simulink library "SimscapeCustomComponents_lib"  (R2025b)
settings: Solver=VariableStepAuto  StartTime=0.0  StopTime=10.0  RelTol=1e-3
undefined symbols (not defined in the file or in its folder): base, baseVdc, capacity, DiscIntNeverNeededParam, ee_sli_rtmsupport, filterInductance, freqeuncy, frequency, gcbh, gflInverter, gfmInverter, iMaxPU, Inertia, initialSOC, plantRating, solar, Ts, ups, Vac, windSystem, windTurbine
libraries: fl_lib x397, nesl_utility x171, eeGeneralControl x85, ee_lib x82, simulink x72, datacenter_lib x68, eeTransforms x38, slpidlib x24, buildingEnergy_lib x20, SimscapeFluids_lib x17, eeSinusoidalMeasurementV2 x8, eePwmGenerator x8
(part 10 of 24)

== system SimscapeCustomComponents_lib/Microgrid and Renewables/Control/Microgrid/Black Start ==
  Enable : Inport  OutDataTypeStr=boolean
  Voltage : Inport  Port=2  OutDataTypeStr=boolean
  Abs : Abs  SaturateOnIntegerOverflow=off
  Constant : Constant  Value=0.05
  Constant1 : Constant  Value=voltageLevel1+voltageLevel2+voltageLevel3
  Data Type Conversion : DataTypeConversion  OutDataTypeStr=double  SaturateOnIntegerOverflow=off  RndMeth=Floor
  Data Type Conversion1 : DataTypeConversion  OutDataTypeStr=boolean  SaturateOnIntegerOverflow=off  RndMeth=Floor
  Delay : Delay  DelayLength=10
  Frequency Reference : Subsystem
  Gain : Gain
  LessThanOrEqual : RelationalOperator  Operator=<=  OutDataTypeStr=boolean  RndMeth=Simplest  InputSameDT=off
  Product : Product
  Subtract : Sum  Inputs=+-
  Voltage Reference : Subsystem
  Status : Outport
  Bus Element Out2 : Outport  Port=2  PortName=BlackStart  Element=Vref
  Bus Element Out3 : Outport  Port=2  PortName=BlackStart  Element=Fref
  Bus Element Out1 : Outport  Port=2  PortName=BlackStart  Element=enableCommand
  wires:
  Voltage Reference/1(VRef) -> Bus Element Out2/1
  Data Type Conversion/1 -> Gain/1
  Data Type Conversion1/1 -> Status/1
  Enable/1 -> Voltage Reference/1(Enable), Data Type Conversion/1
  Delay/1 -> Product/1
  Abs/1 -> LessThanOrEqual/1
  Constant1/1 -> Subtract/2
  Product/1 -> Data Type Conversion1/1
  Voltage/1 -> Subtract/1
  Constant/1 -> LessThanOrEqual/2
  LessThanOrEqual/1 -> Product/2
  Frequency Reference/1(FRef) -> Bus Element Out3/1
  Subtract/1 -> Abs/1
  Gain/1 -> Bus Element Out1/1, Delay/1

== system SimscapeCustomComponents_lib/Microgrid and Renewables/Control/Microgrid/PlannedIslanding ==
  Enable : Inport
  P : Inport  Port=2
  Q : Inport  Port=3
  Data Type Conversion : DataTypeConversion  OutDataTypeStr=double  SaturateOnIntegerOverflow=off  RndMeth=Floor
  Logical Operator : Logic  AllPortsSameDT=off  OutDataTypeStr=boolean
  PID Frequency : slpidlib/PID Controller  Controller=PI  Form=Parallel  TimeDomain=Discrete-time  UseExternalTs=off  SampleTime=Ts  IntegratorMethod=Forward Euler  FilterMethod=Forward Euler  ControllerParametersSource=internal  P=KpPPlannedIsland  I=KiPPlannedIsland  UseKiTs=off  D=0  UseExternalDerivativeSource=off  N=100  UseFilter=on  TunerSelectOption=Frequency Response Based  InitialConditionSource=internal  InitialConditionForIntegrator=0  InitialConditionForFilter=0  DifferentiatorICPrevScaledInput=0  ExternalReset=none  TrackingMode=off  Kt=1  LimitOutput=off  SatLimitsSource=internal  UpperSaturationLimit=0.05  LowerSaturationLimit=-0.05  LinearizeAsGain=on  AntiWindupMode=clamping  Kb=1  LimitIntegrator=off  UpperIntegratorSaturationLimit=inf  LowerIntegratorSaturationLimit=-inf  POutMin=[]  POutMax=[]  IOutMin=[]  IOutMax=[]  DOutMin=[]  DOutMax=[]  NOutMin=[]  NOutMax=[]  SumOutMin=[]  SumOutMax=[]  SaturationOutMin=[]  SaturationOutMax=[]  PParamMin=[]  PParamMax=[]  IParamMin=[]  IParamMax=[]  DParamMin=[]  DParamMax=[]  NParamMin=[]  NParamMax=[]  KbParamMin=[]  KbParamMax=[]  KtParamMin=[]  KtParamMax=[]  KbOutMin=[]  KbOutMax=[]  KtOutMin=[]  KtOutMax=[]  IntegratorOutMin=[]  IntegratorOutMax=[]  FilterOutMin=[]  FilterOutMax=[]  SumI1OutMin=[]  SumI1OutMax=[]  SumI2OutMin=[]  SumI2OutMax=[]  SumI3OutMin=[]  SumI3OutMax=[]  SumI4OutMin=[]  SumI4OutMax=[]  SumDOutMin=[]  SumDOutMax=[]  DifferentiatorOutMin=[]  DifferentiatorOutMax=[]  FilterDiffOutCoefMin=[]  FilterDiffOutCoefMax=[]  ReciprocalOutMin=[]  ReciprocalOutMax=[]  SumDenOutMin=[]  SumDenOutMax=[]  SumNumOutMin=[]  SumNumOutMax=[]  DivideOutMin=[]  DivideOutMax=[]  UdiffTsProdOutMin=[]  UdiffTsProdOutMax=[]  NTsProdOutMin=[]  NTsProdOutMax=[]  UintegralTsProdOutMin=[]  UintegralTsProdOutMax=[]  UngainTsProdOutMin=[]  UngainTsProdOutMax=[]  ClampingZeroOutDataTypeStr=Inherit: Inherit via back propagation  ClampingZeroOutMin=[]  ClampingZeroOutMax=[]  FilterDenConstantOutDataTypeStr=Inherit: Inherit via back propagation  FilterDenConstantOutMin=[]  FilterDenConstantOutMax=[]  PCopyOutDataTypeStr=Inherit: Inherit via back propagation  PCopyOutMin=[]  PCopyOutMax=[]  NCopyOutDataTypeStr=Inherit: Inherit via back propagation  NCopyOutMin=[]  NCopyOutMax=[]  IntegratorContinuousStateAttributes=''  IntegratorStateMustResolveToSignalObject=off  IntegratorRTWStateStorageClass=Auto  FilterContinuousStateAttributes=''  FilterStateMustResolveToSignalObject=off  FilterRTWStateStorageClass=Auto  ParallelPVariant=InternalParameters  IdealPVariant=Disabled  IVariant=InternalParameters  DVariant=Disabled  IntegratorVariant=Discrete  SatVariant=Disabled  AWVariant=Passthrough  PCopyVariant=Disabled  TRVariant=Disabled  FdbkBlocksVariant=Forward  IdealPFdbkVariant=Disabled  SatFdbkVariant=Disabled  DerivativeFilterVariant=Disabled  NVariant=Disabled  NCopyVariant=Disabled_SignalSpec  FilterICVariant=Disabled  IntegratorICVariant=InternalICs  ExternalResetVariant=Disabled  TRSumVariant=Passthrough  SumFdbkVariant=Disabled  SumVariant=Sum_PI  TsampFilterVariant=InternalTs  TsampNgainVariant=Passthrough  TsampIntegralVariant=Disabled_SignalSpec  ExternalSaturationOutDataTypeStr=Inherit: Same as second input  DerivativeSourceVariant=Disabled  PreIntVariant=InternalPreInt
  PID voltage : slpidlib/PID Controller  Controller=PI  Form=Parallel  TimeDomain=Discrete-time  UseExternalTs=off  SampleTime=Ts  IntegratorMethod=Forward Euler  FilterMethod=Forward Euler  ControllerParametersSource=internal  P=KpQPlannedIsland  I=KiQPlannedIsland  UseKiTs=off  D=0  UseExternalDerivativeSource=off  N=100  UseFilter=on  TunerSelectOption=Frequency Response Based  InitialConditionSource=internal  InitialConditionForIntegrator=0  InitialConditionForFilter=0  DifferentiatorICPrevScaledInput=0  ExternalReset=none  TrackingMode=off  Kt=1  LimitOutput=off  SatLimitsSource=internal  UpperSaturationLimit=0.05  LowerSaturationLimit=-0.05  LinearizeAsGain=on  AntiWindupMode=clamping  Kb=1  LimitIntegrator=off  UpperIntegratorSaturationLimit=inf  LowerIntegratorSaturationLimit=-inf  POutMin=[]  POutMax=[]  IOutMin=[]  IOutMax=[]  DOutMin=[]  DOutMax=[]  NOutMin=[]  NOutMax=[]  SumOutMin=[]  SumOutMax=[]  SaturationOutMin=[]  SaturationOutMax=[]  PParamMin=[]  PParamMax=[]  IParamMin=[]  IParamMax=[]  DParamMin=[]  DParamMax=[]  NParamMin=[]  NParamMax=[]  KbParamMin=[]  KbParamMax=[]  KtParamMin=[]  KtParamMax=[]  KbOutMin=[]  KbOutMax=[]  KtOutMin=[]  KtOutMax=[]  IntegratorOutMin=[]  IntegratorOutMax=[]  FilterOutMin=[]  FilterOutMax=[]  SumI1OutMin=[]  SumI1OutMax=[]  SumI2OutMin=[]  SumI2OutMax=[]  SumI3OutMin=[]  SumI3OutMax=[]  SumI4OutMin=[]  SumI4OutMax=[]  SumDOutMin=[]  SumDOutMax=[]  DifferentiatorOutMin=[]  DifferentiatorOutMax=[]  FilterDiffOutCoefMin=[]  FilterDiffOutCoefMax=[]  ReciprocalOutMin=[]  ReciprocalOutMax=[]  SumDenOutMin=[]  SumDenOutMax=[]  SumNumOutMin=[]  SumNumOutMax=[]  DivideOutMin=[]  DivideOutMax=[]  UdiffTsProdOutMin=[]  UdiffTsProdOutMax=[]  NTsProdOutMin=[]  NTsProdOutMax=[]  UintegralTsProdOutMin=[]  UintegralTsProdOutMax=[]  UngainTsProdOutMin=[]  UngainTsProdOutMax=[]  ClampingZeroOutDataTypeStr=Inherit: Inherit via back propagation  ClampingZeroOutMin=[]  ClampingZeroOutMax=[]  FilterDenConstantOutDataTypeStr=Inherit: Inherit via back propagation  FilterDenConstantOutMin=[]  FilterDenConstantOutMax=[]  PCopyOutDataTypeStr=Inherit: Inherit via back propagation  PCopyOutMin=[]  PCopyOutMax=[]  NCopyOutDataTypeStr=Inherit: Inherit via back propagation  NCopyOutMin=[]  NCopyOutMax=[]  IntegratorContinuousStateAttributes=''  IntegratorStateMustResolveToSignalObject=off  IntegratorRTWStateStorageClass=Auto  FilterContinuousStateAttributes=''  FilterStateMustResolveToSignalObject=off  FilterRTWStateStorageClass=Auto  ParallelPVariant=InternalParameters  IdealPVariant=Disabled  IVariant=InternalParameters  DVariant=Disabled  IntegratorVariant=Discrete  SatVariant=Disabled  AWVariant=Passthrough  PCopyVariant=Disabled  TRVariant=Disabled  FdbkBlocksVariant=Forward  IdealPFdbkVariant=Disabled  SatFdbkVariant=Disabled  DerivativeFilterVariant=Disabled  NVariant=Disabled  NCopyVariant=Disabled_SignalSpec  FilterICVariant=Disabled  IntegratorICVariant=InternalICs  ExternalResetVariant=Disabled  TRSumVariant=Passthrough  SumFdbkVariant=Disabled  SumVariant=Sum_PI  TsampFilterVariant=InternalTs  TsampNgainVariant=Passthrough  TsampIntegralVariant=Disabled_SignalSpec  ExternalSaturationOutDataTypeStr=Inherit: Same as second input  DerivativeSourceVariant=Disabled  PreIntVariant=InternalPreInt
  Planned Island Time Delay : Subsystem
  Product{,1..3} (4 alike) : Product
  Scope : Scope  NumInputPorts=2
      settings: ActiveDisplayYMinimum=-1  ActiveDisplayYMaximum=1  DataLoggingVariableName=ScopeData35
  Scope1 : Scope  NumInputPorts=2
      settings: ActiveDisplayYMinimum=-1.6827967094302978  ActiveDisplayYMaximum=1.1685546180291482  DataLoggingVariableName=ScopeData36
  Subsystem : Subsystem
  Subsystem1 : Subsystem
  Status : Outport
  Bus Element Out : Outport  Port=2  PortName=PlannedIslanding  Element=enableCommand
  BusElementOut : Outport  Port=2  PortName=PlannedIslanding  Element=activePower
  BusElementOut1 : Outport  Port=2  PortName=PlannedIslanding  Element=reactivePower
  BusElementOut2 : Outport  Port=2  PortName=PlannedIslanding  Element=status
  wires:
  Product1/1 -> Subsystem/1(AVTIVE POWER ERROR), PID Frequency/1
  Product3/1 -> Logical Operator/2
  PID voltage/1 -> Scope/2, BusElementOut1/1
  [plannedIslanding] -> Product3/1
  [plannedIslanding] -> Planned Island Time Delay/2(In2)
  [plannedIslanding] -> Product/1
  PID Frequency/1 -> BusElementOut/1, Scope/1
  Planned Island Time Delay/1(Status) -> BusElementOut2/1, Status/1
  Product/1 -> Logical Operator/1
  Q/1 -> Scope1/2, Product2/2
  Subsystem1/1(Out1) -> Product3/2
  [plannedIslanding] -> Product1/2, Product2/1
  Subsystem/1(Out1) -> Product/2
  P/1 -> Scope1/1, Product1/1
  Logical Operator/1 -> Planned Island Time Delay/1(In1)
  Enable/1 -> Data Type Conversion/1
  Product2/1 -> PID voltage/1, Subsystem1/1(REACTIVEPOWER ERROR)
  Data Type Conversion/1 -> Bus Element Out/1, [plannedIslanding]
  ? -> ?

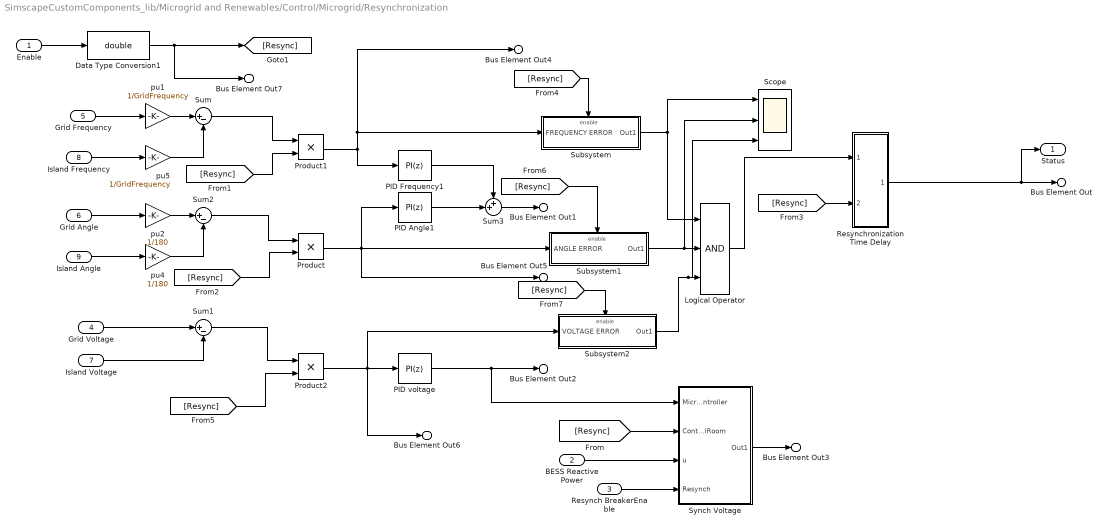
== system SimscapeCustomComponents_lib/Microgrid and Renewables/Control/Microgrid/Resynchronization ==
  Enable : Inport  OutDataTypeStr=double
  BESS Reactive Power : Inport  Port=2
  Resynch BreakerEnable : Inport  Port=3
  Grid Voltage : Inport  Port=4
  Grid Frequency : Inport  Port=5
  Grid Angle : Inport  Port=6
  Island Voltage : Inport  Port=7
  Island Frequency : Inport  Port=8
  Island Angle : Inport  Port=9
  Data Type Conversion1 : DataTypeConversion  OutDataTypeStr=double  SaturateOnIntegerOverflow=off  RndMeth=Floor
  Logical Operator : Logic  Inputs=3  AllPortsSameDT=off  OutDataTypeStr=boolean
  PID Angle1 : slpidlib/PID Controller  Controller=PI  Form=Parallel  TimeDomain=Discrete-time  UseExternalTs=off  SampleTime=Ts  IntegratorMethod=Forward Euler  FilterMethod=Forward Euler  ControllerParametersSource=internal  P=KpAngResynch  I=KiAngResynch  UseKiTs=off  D=0  UseExternalDerivativeSource=off  N=100  UseFilter=on  TunerSelectOption=Frequency Response Based  InitialConditionSource=internal  InitialConditionForIntegrator=0  InitialConditionForFilter=0  DifferentiatorICPrevScaledInput=0  ExternalReset=none  TrackingMode=off  Kt=1  LimitOutput=off  SatLimitsSource=internal  UpperSaturationLimit=0.5  LowerSaturationLimit=-0.5  LinearizeAsGain=on  AntiWindupMode=clamping  Kb=1  LimitIntegrator=off  UpperIntegratorSaturationLimit=inf  LowerIntegratorSaturationLimit=-inf  POutMin=[]  POutMax=[]  IOutMin=[]  IOutMax=[]  DOutMin=[]  DOutMax=[]  NOutMin=[]  NOutMax=[]  SumOutMin=[]  SumOutMax=[]  SaturationOutMin=[]  SaturationOutMax=[]  PParamMin=[]  PParamMax=[]  IParamMin=[]  IParamMax=[]  DParamMin=[]  DParamMax=[]  NParamMin=[]  NParamMax=[]  KbParamMin=[]  KbParamMax=[]  KtParamMin=[]  KtParamMax=[]  KbOutMin=[]  KbOutMax=[]  KtOutMin=[]  KtOutMax=[]  IntegratorOutMin=[]  IntegratorOutMax=[]  FilterOutMin=[]  FilterOutMax=[]  SumI1OutMin=[]  SumI1OutMax=[]  SumI2OutMin=[]  SumI2OutMax=[]  SumI3OutMin=[]  SumI3OutMax=[]  SumI4OutMin=[]  SumI4OutMax=[]  SumDOutMin=[]  SumDOutMax=[]  DifferentiatorOutMin=[]  DifferentiatorOutMax=[]  FilterDiffOutCoefMin=[]  FilterDiffOutCoefMax=[]  ReciprocalOutMin=[]  ReciprocalOutMax=[]  SumDenOutMin=[]  SumDenOutMax=[]  SumNumOutMin=[]  SumNumOutMax=[]  DivideOutMin=[]  DivideOutMax=[]  UdiffTsProdOutMin=[]  UdiffTsProdOutMax=[]  NTsProdOutMin=[]  NTsProdOutMax=[]  UintegralTsProdOutMin=[]  UintegralTsProdOutMax=[]  UngainTsProdOutMin=[]  UngainTsProdOutMax=[]  ClampingZeroOutDataTypeStr=Inherit: Inherit via back propagation  ClampingZeroOutMin=[]  ClampingZeroOutMax=[]  FilterDenConstantOutDataTypeStr=Inherit: Inherit via back propagation  FilterDenConstantOutMin=[]  FilterDenConstantOutMax=[]  PCopyOutDataTypeStr=Inherit: Inherit via back propagation  PCopyOutMin=[]  PCopyOutMax=[]  NCopyOutDataTypeStr=Inherit: Inherit via back propagation  NCopyOutMin=[]  NCopyOutMax=[]  IntegratorContinuousStateAttributes=''  IntegratorStateMustResolveToSignalObject=off  IntegratorRTWStateStorageClass=Auto  FilterContinuousStateAttributes=''  FilterStateMustResolveToSignalObject=off  FilterRTWStateStorageClass=Auto  ParallelPVariant=InternalParameters  IdealPVariant=Disabled  IVariant=InternalParameters  DVariant=Disabled  IntegratorVariant=Discrete  SatVariant=Disabled  AWVariant=Passthrough  PCopyVariant=Disabled  TRVariant=Disabled  FdbkBlocksVariant=Forward  IdealPFdbkVariant=Disabled  SatFdbkVariant=Disabled  DerivativeFilterVariant=Disabled  NVariant=Disabled  NCopyVariant=Disabled_SignalSpec  FilterICVariant=Disabled  IntegratorICVariant=InternalICs  ExternalResetVariant=Disabled  TRSumVariant=Passthrough  SumFdbkVariant=Disabled  SumVariant=Sum_PI  TsampFilterVariant=InternalTs  TsampNgainVariant=Passthrough  TsampIntegralVariant=Disabled_SignalSpec  ExternalSaturationOutDataTypeStr=Inherit: Same as second input  DerivativeSourceVariant=Disabled  PreIntVariant=InternalPreInt
  PID Frequency1 : slpidlib/PID Controller  Controller=PI  Form=Parallel  TimeDomain=Discrete-time  UseExternalTs=off  SampleTime=Ts  IntegratorMethod=Forward Euler  FilterMethod=Forward Euler  ControllerParametersSource=internal  P=KpFreResynch  I=KiFreResynch  UseKiTs=off  D=0  UseExternalDerivativeSource=off  N=100  UseFilter=on  TunerSelectOption=Frequency Response Based  InitialConditionSource=internal  InitialConditionForIntegrator=0  InitialConditionForFilter=0  DifferentiatorICPrevScaledInput=0  ExternalReset=none  TrackingMode=off  Kt=1  LimitOutput=off  SatLimitsSource=internal  UpperSaturationLimit=0.05  LowerSaturationLimit=-0.05  LinearizeAsGain=on  AntiWindupMode=clamping  Kb=1  LimitIntegrator=off  UpperIntegratorSaturationLimit=inf  LowerIntegratorSaturationLimit=-inf  POutMin=[]  POutMax=[]  IOutMin=[]  IOutMax=[]  DOutMin=[]  DOutMax=[]  NOutMin=[]  NOutMax=[]  SumOutMin=[]  SumOutMax=[]  SaturationOutMin=[]  SaturationOutMax=[]  PParamMin=[]  PParamMax=[]  IParamMin=[]  IParamMax=[]  DParamMin=[]  DParamMax=[]  NParamMin=[]  NParamMax=[]  KbParamMin=[]  KbParamMax=[]  KtParamMin=[]  KtParamMax=[]  KbOutMin=[]  KbOutMax=[]  KtOutMin=[]  KtOutMax=[]  IntegratorOutMin=[]  IntegratorOutMax=[]  FilterOutMin=[]  FilterOutMax=[]  SumI1OutMin=[]  SumI1OutMax=[]  SumI2OutMin=[]  SumI2OutMax=[]  SumI3OutMin=[]  SumI3OutMax=[]  SumI4OutMin=[]  SumI4OutMax=[]  SumDOutMin=[]  SumDOutMax=[]  DifferentiatorOutMin=[]  DifferentiatorOutMax=[]  FilterDiffOutCoefMin=[]  FilterDiffOutCoefMax=[]  ReciprocalOutMin=[]  ReciprocalOutMax=[]  SumDenOutMin=[]  SumDenOutMax=[]  SumNumOutMin=[]  SumNumOutMax=[]  DivideOutMin=[]  DivideOutMax=[]  UdiffTsProdOutMin=[]  UdiffTsProdOutMax=[]  NTsProdOutMin=[]  NTsProdOutMax=[]  UintegralTsProdOutMin=[]  UintegralTsProdOutMax=[]  UngainTsProdOutMin=[]  UngainTsProdOutMax=[]  ClampingZeroOutDataTypeStr=Inherit: Inherit via back propagation  ClampingZeroOutMin=[]  ClampingZeroOutMax=[]  FilterDenConstantOutDataTypeStr=Inherit: Inherit via back propagation  FilterDenConstantOutMin=[]  FilterDenConstantOutMax=[]  PCopyOutDataTypeStr=Inherit: Inherit via back propagation  PCopyOutMin=[]  PCopyOutMax=[]  NCopyOutDataTypeStr=Inherit: Inherit via back propagation  NCopyOutMin=[]  NCopyOutMax=[]  IntegratorContinuousStateAttributes=''  IntegratorStateMustResolveToSignalObject=off  IntegratorRTWStateStorageClass=Auto  FilterContinuousStateAttributes=''  FilterStateMustResolveToSignalObject=off  FilterRTWStateStorageClass=Auto  ParallelPVariant=InternalParameters  IdealPVariant=Disabled  IVariant=InternalParameters  DVariant=Disabled  IntegratorVariant=Discrete  SatVariant=Disabled  AWVariant=Passthrough  PCopyVariant=Disabled  TRVariant=Disabled  FdbkBlocksVariant=Forward  IdealPFdbkVariant=Disabled  SatFdbkVariant=Disabled  DerivativeFilterVariant=Disabled  NVariant=Disabled  NCopyVariant=Disabled_SignalSpec  FilterICVariant=Disabled  IntegratorICVariant=InternalICs  ExternalResetVariant=Disabled  TRSumVariant=Passthrough  SumFdbkVariant=Disabled  SumVariant=Sum_PI  TsampFilterVariant=InternalTs  TsampNgainVariant=Passthrough  TsampIntegralVariant=Disabled_SignalSpec  ExternalSaturationOutDataTypeStr=Inherit: Same as second input  DerivativeSourceVariant=Disabled  PreIntVariant=InternalPreInt
  PID voltage : slpidlib/PID Controller  Controller=PI  Form=Parallel  TimeDomain=Discrete-time  UseExternalTs=off  SampleTime=Ts  IntegratorMethod=Forward Euler  FilterMethod=Forward Euler  ControllerParametersSource=internal  P=KpVolResynch  I=KiVolResynch  UseKiTs=off  D=0  UseExternalDerivativeSource=off  N=100  UseFilter=on  TunerSelectOption=Frequency Response Based  InitialConditionSource=internal  InitialConditionForIntegrator=1  InitialConditionForFilter=0  DifferentiatorICPrevScaledInput=0  ExternalReset=none  TrackingMode=off  Kt=1  LimitOutput=off  SatLimitsSource=internal  UpperSaturationLimit=1.5  LowerSaturationLimit=-0.05  LinearizeAsGain=on  AntiWindupMode=clamping  Kb=1  LimitIntegrator=off  UpperIntegratorSaturationLimit=inf  LowerIntegratorSaturationLimit=-inf  POutMin=[]  POutMax=[]  IOutMin=[]  IOutMax=[]  DOutMin=[]  DOutMax=[]  NOutMin=[]  NOutMax=[]  SumOutMin=[]  SumOutMax=[]  SaturationOutMin=[]  SaturationOutMax=[]  PParamMin=[]  PParamMax=[]  IParamMin=[]  IParamMax=[]  DParamMin=[]  DParamMax=[]  NParamMin=[]  NParamMax=[]  KbParamMin=[]  KbParamMax=[]  KtParamMin=[]  KtParamMax=[]  KbOutMin=[]  KbOutMax=[]  KtOutMin=[]  KtOutMax=[]  IntegratorOutMin=[]  IntegratorOutMax=[]  FilterOutMin=[]  FilterOutMax=[]  SumI1OutMin=[]  SumI1OutMax=[]  SumI2OutMin=[]  SumI2OutMax=[]  SumI3OutMin=[]  SumI3OutMax=[]  SumI4OutMin=[]  SumI4OutMax=[]  SumDOutMin=[]  SumDOutMax=[]  DifferentiatorOutMin=[]  DifferentiatorOutMax=[]  FilterDiffOutCoefMin=[]  FilterDiffOutCoefMax=[]  ReciprocalOutMin=[]  ReciprocalOutMax=[]  SumDenOutMin=[]  SumDenOutMax=[]  SumNumOutMin=[]  SumNumOutMax=[]  DivideOutMin=[]  DivideOutMax=[]  UdiffTsProdOutMin=[]  UdiffTsProdOutMax=[]  NTsProdOutMin=[]  NTsProdOutMax=[]  UintegralTsProdOutMin=[]  UintegralTsProdOutMax=[]  UngainTsProdOutMin=[]  UngainTsProdOutMax=[]  ClampingZeroOutDataTypeStr=Inherit: Inherit via back propagation  ClampingZeroOutMin=[]  ClampingZeroOutMax=[]  FilterDenConstantOutDataTypeStr=Inherit: Inherit via back propagation  FilterDenConstantOutMin=[]  FilterDenConstantOutMax=[]  PCopyOutDataTypeStr=Inherit: Inherit via back propagation  PCopyOutMin=[]  PCopyOutMax=[]  NCopyOutDataTypeStr=Inherit: Inherit via back propagation  NCopyOutMin=[]  NCopyOutMax=[]  IntegratorContinuousStateAttributes=''  IntegratorStateMustResolveToSignalObject=off  IntegratorRTWStateStorageClass=Auto  FilterContinuousStateAttributes=''  FilterStateMustResolveToSignalObject=off  FilterRTWStateStorageClass=Auto  ParallelPVariant=InternalParameters  IdealPVariant=Disabled  IVariant=InternalParameters  DVariant=Disabled  IntegratorVariant=Discrete  SatVariant=Disabled  AWVariant=Passthrough  PCopyVariant=Disabled  TRVariant=Disabled  FdbkBlocksVariant=Forward  IdealPFdbkVariant=Disabled  SatFdbkVariant=Disabled  DerivativeFilterVariant=Disabled  NVariant=Disabled  NCopyVariant=Disabled_SignalSpec  FilterICVariant=Disabled  IntegratorICVariant=InternalICs  ExternalResetVariant=Disabled  TRSumVariant=Passthrough  SumFdbkVariant=Disabled  SumVariant=Sum_PI  TsampFilterVariant=InternalTs  TsampNgainVariant=Passthrough  TsampIntegralVariant=Disabled_SignalSpec  ExternalSaturationOutDataTypeStr=Inherit: Same as second input  DerivativeSourceVariant=Disabled  PreIntVariant=InternalPreInt
  Product : Product
  Product1 : Product
  Product2 : Product
  Resynchronization Time Delay : Subsystem
  Scope : Scope  NumInputPorts=3
      settings: ActiveDisplayYMinimum=-1  ActiveDisplayYMaximum=1  DataLoggingVariableName=ScopeData40
  Subsystem : Subsystem
  Subsystem1 : Subsystem
  Subsystem2 : Subsystem
  Sum : Sum  Inputs=|+-
  Sum1 : Sum  Inputs=|+-
  Sum2 : Sum  Inputs=|+-
  Sum3 : Sum  Inputs=++|
  Synch Voltage : Subsystem
  pu1 : Gain  Gain=1/GridFrequency
  pu2 : Gain  Gain=1/180
  pu4 : Gain  Gain=1/180
  pu5 : Gain  Gain=1/GridFrequency
  Status : Outport
  Bus Element Out : Outport  Port=2  PortName=Resync  Element=status
  Bus Element Out1 : Outport  Port=2  PortName=Resync  Element=synchFrequency
  Bus Element Out2 : Outport  Port=2  PortName=Resync  Element=synchVoltage
  Bus Element Out3 : Outport  Port=2  PortName=Resync  Element=synchVoltagedpr
  Bus Element Out4 : Outport  Port=2  PortName=Resync  Element=frequencyerror
  Bus Element Out5 : Outport  Port=2  PortName=Resync  Element=phasError
  Bus Element Out6 : Outport  Port=2  PortName=Resync  Element=voltageMagError
  Bus Element Out7 : Outport  Port=2  PortName=Resync  Element=enableCommand
  wires:
  [Resync] -> Subsystem1/Enable
  [Resync] -> Product/2
  [Resync] -> Subsystem/Enable
  PID voltage/1 -> Synch Voltage/1(MicrogridController), Bus Element Out2/1
  Sum/1 -> Product1/1
  Sum3/1 -> Bus Element Out1/1
  Enable/1 -> Data Type Conversion1/1
  Sum1/1 -> Product2/1
  Synch Voltage/1(Out1) -> Bus Element Out3/1
  [Resync] -> Subsystem2/Enable
  Subsystem1/1(Out1) -> Scope/2, Logical Operator/2
  Subsystem2/1(Out1) -> Scope/3, Logical Operator/3
  [Resync] -> Synch Voltage/2(ControlRoom)
  Logical Operator/1 -> Resynchronization Time Delay/1(In1)
  [Resync] -> Resynchronization Time Delay/2(In2)
  [Resync] -> Product2/2
  pu5/1 -> Sum/2
  Resynchronization Time Delay/1(MGController) -> Status/1, Bus Element Out/1
  Subsystem/1(Out1) -> Scope/1, Logical Operator/1
  Product/1 -> PID Angle1/1, Subsystem1/1(ANGLE ERROR), Bus Element Out5/1
  Grid Frequency/1 -> pu1/1
  Grid Angle/1 -> pu2/1
  [Resync] -> Product1/2
  Island Angle/1 -> pu4/1
  Grid Voltage/1 -> Sum1/1
  Product2/1 -> Subsystem2/1(VOLTAGE ERROR), Bus Element Out6/1, PID voltage/1
  Data Type Conversion1/1 -> [Resync], Bus Element Out7/1
  pu2/1 -> Sum2/1
  Island Frequency/1 -> pu5/1
  PID Angle1/1 -> Sum3/2
  BESS Reactive Power/1 -> Synch Voltage/3(u)
  pu4/1 -> Sum2/2
  Sum2/1 -> Product/1
  Product1/1 -> PID Frequency1/1, Subsystem/1(FREQUENCY ERROR), Bus Element Out4/1
  Island Voltage/1 -> Sum1/2
  Resynch BreakerEnable/1 -> Synch Voltage/4(Resynch)
  pu1/1 -> Sum/1
  PID Frequency1/1 -> Sum3/1

== system SimscapeCustomComponents_lib/Microgrid and Renewables/Control/Renewables/Power Reference Controller ==
  Iabc : Inport
  Vabc : Inport  Port=2
  Pref : Inport  Port=3
  Qref : Inport  Port=4
  Constant : Constant  Value=10
  PLL & Measurements : Subsystem
      mask Display: image('$imagefile'); % Use "Edit Image" on toolstrip to change.
  Power Reference Controller : Subsystem  mask{mp=0, mv=0, P=Real power, MVA=MVA, zbase=Vac^2/(MVA), L=L, Imax=Imax, Td=1e-3, Kpic=Kpic, Kiic=Kiic, Kd=0}
      mask prompts: mp "Real power droop cofficient"; mv "Reactive power droop cofficient"; P "Priority mode"; MVA "Base Power (V*A)"; zbase "Base Impedance (Ohm)"; L "Filter Inductance (H)"; Imax "Inverter current limit (pu)"; Td "Sensor time delay (s)"; Kpic "Proportional gain"; Kiic "Integral gain"; Kd "Derevative gain"
      mask TypeOptions P: Real power  | Reactive power
      mask DialogControl Container4 Prompt: General
      mask DialogControl Container5 Prompt: Current Controller
  mabc : Outport
  wires:
  Qref/1 -> Power Reference Controller/4(Qref)
  Constant/1 -> Power Reference Controller/2(LVRT_iq)
  Vabc/1 -> PLL & Measurements/1(V)
  Iabc/1 -> PLL & Measurements/2(I)
  Power Reference Controller/1(m_abc) -> mabc/1
  PLL & Measurements/1(VIbus) -> Power Reference Controller/1(VIbus)
  Pref/1 -> Power Reference Controller/3(Pref)

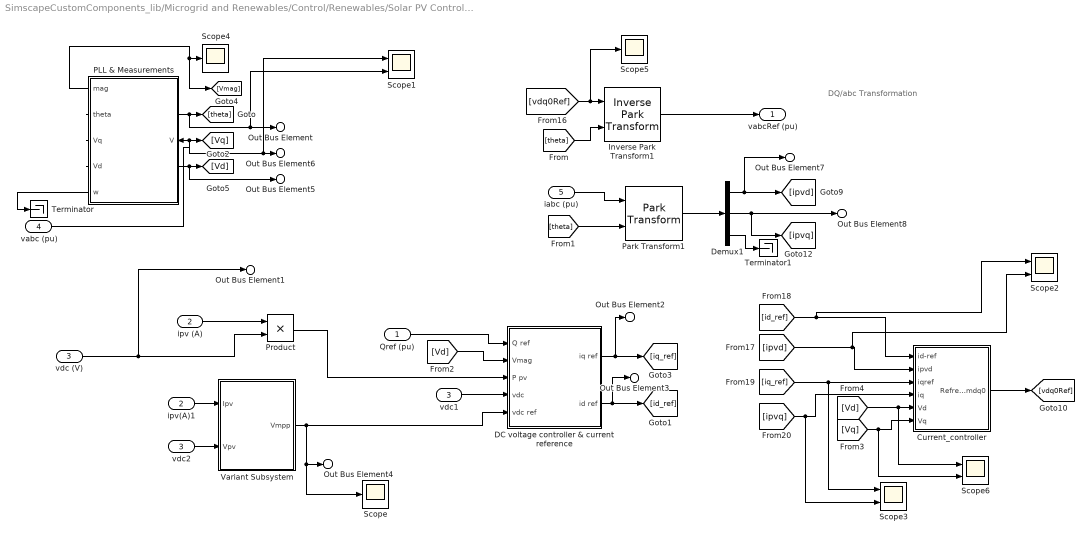
== system SimscapeCustomComponents_lib/Microgrid and Renewables/Control/Renewables/Solar PV Controller ==
  note: DQ/abc Transformation
  Qref (pu) : Inport
  ipv (A) : Inport  Port=2
  vdc (V) : Inport  Port=3
  vabc (pu) : Inport  Port=4
  iabc (pu) : Inport  Port=5
  Current_controller : Subsystem  SystemSampleTime=sampleTime
  DC voltage controller & current reference : Subsystem  SystemSampleTime=sampleTime
  Demux1 : Demux  Outputs=3
  Inverse Park Transform1 : eeTransforms/Inverse Park Transform  AxisAlignment=Q-axis  PowerInvariant=off
  PLL & Measurements : Subsystem
  Park Transform1 : eeTransforms/Park Transform  AxisAlignment=Q-axis  PowerInvariant=off
  Product : Product
  Scope : Scope
      settings: ActiveDisplayYMinimum=719.47133  ActiveDisplayYMaximum=1441.72759  DataLoggingVariableName=ScopeData5
  Scope{1..3,6} (4 alike) : Scope  NumInputPorts=2
      Scope1 settings: ActiveDisplayYMinimum=-0.55297  ActiveDisplayYMaximum=0.65726  DataLoggingVariableName=ScopeData6
      Scope2 settings: ActiveDisplayYMinimum=0.74203  ActiveDisplayYMaximum=1.09578
      Scope3 settings: ActiveDisplayYMinimum=-1  ActiveDisplayYMaximum=1
      Scope6 settings: ActiveDisplayYMinimum=0.97205  ActiveDisplayYMaximum=1.00522  DataLoggingVariableName=ScopeData6
  Scope4 : Scope
      settings: ActiveDisplayYMinimum=-0.12504  ActiveDisplayYMaximum=1.12534
  Scope5 : Scope
      settings: ActiveDisplayYMinimum=-0.12621  ActiveDisplayYMaximum=1.13592
  Terminator : Terminator
  Terminator1 : Terminator
  Variant Subsystem : Subsystem  Variant=on  VariantControlMode=label  LabelModeActiveChoice=Perturb and observe (P&O)
  ipv(A)1 : InportShadow  Port=2
  vdc1 : InportShadow  Port=3
  vdc2 : InportShadow  Port=3
  vabcRef (pu) : Outport
  Out Bus Element : Outport  Port=2  PortName=visualization  Element=theta [rad]
  Out Bus Element1 : Outport  Port=2  PortName=visualization  Element=vdc [Volts]
  Out Bus Element2 : Outport  Port=2  PortName=visualization  Element=iq ref [pu]
  Out Bus Element3 : Outport  Port=2  PortName=visualization  Element=id ref [pu]
  Out Bus Element4 : Outport  Port=2  PortName=visualization  Element=vdc ref [Volts]
  Out Bus Element5 : Outport  Port=2  PortName=visualization  Element=Vd [pu]
  Out Bus Element6 : Outport  Port=2  PortName=visualization  Element=Vq [pu]
  Out Bus Element7 : Outport  Port=2  PortName=visualization  Element=id [pu]
  Out Bus Element8 : Outport  Port=2  PortName=visualization  Element=iq [pu]
  wires:
  [Vq] -> Current_controller/6(Vq), Scope6/2
  Current_controller/1(Refrence_mdq0) -> [vdq0Ref]
  Demux1/2 -> Out Bus Element8/1, [ipvq]
  Inverse Park Transform1/1 -> vabcRef (pu)/1
  Demux1/1 -> Out Bus Element7/1, [ipvd]
  Demux1/3 -> Terminator1/1
  [vdq0Ref] -> Inverse Park Transform1/1, Scope5/1
  Park Transform1/1 -> Demux1/1
  [id_ref] -> Current_controller/1(id-ref), Scope2/1
  [Vd] -> Current_controller/5(Vd), Scope6/1
  [iq_ref] -> Current_controller/3(iqref), Scope3/1
  [ipvq] -> Current_controller/4(iq), Scope3/2
  [theta] -> Park Transform1/2
  [theta] -> Inverse Park Transform1/2
  [ipvd] -> Current_controller/2(ipvd), Scope2/2
  iabc (pu)/1 -> Park Transform1/1
  [Vd] -> DC voltage controller & current reference/2(Vmag)
  DC voltage controller & current reference/1(iq ref) -> Out Bus Element2/1, [iq_ref]
  DC voltage controller & current reference/2(id ref) -> Out Bus Element3/1, [id_ref]
  Qref (pu)/1 -> DC voltage controller & current reference/1(Q ref)
  vdc (V)/1 -> Out Bus Element1/1, Product/2
  Product/1 -> DC voltage controller & current reference/3(P pv)
  PLL & Measurements/3(Vq) -> Out Bus Element6/1, Scope1/1, [Vq]
  PLL & Measurements/1(mag) -> [Vmag], Scope4/1
  PLL & Measurements/4(Vd) -> Out Bus Element5/1, [Vd]
  vabc (pu)/1 -> PLL & Measurements/1(V)
  vdc1/1 -> DC voltage controller & current reference/4(vdc)
  Variant Subsystem/1(Vmpp) -> Out Bus Element4/1, Scope/1, DC voltage controller & current reference/5(vdc ref)
  PLL & Measurements/5(w) -> Terminator/1
  ipv (A)/1 -> Product/1
  vdc2/1 -> Variant Subsystem/2(Vpv)
  ipv(A)1/1 -> Variant Subsystem/1(Ipv)
  PLL & Measurements/2(theta) -> Out Bus Element/1, Scope1/2, [theta]

== system SimscapeCustomComponents_lib/Microgrid and Renewables/Control/Renewables/Wind Controller ==
  iPMSM : Inport
  w : Inport  Port=2
  theta : Inport  Port=3
  vdc : Inport  Port=4
  Wind speed : Inport  Port=5
  LVRT : Inport  Port=6
  QRef : Inport  Port=7
  VIbus : Inport  Port=8
  Machine Converter Control : Subsystem
  Wind Grid-side Converter Controller : Subsystem
  Chopper Control : Outport
  SM converter control : Outport  Port=2
  m_abc : Outport  Port=3
  wires:
  LVRT/1 -> Wind Grid-side Converter Controller/3(LVRT)
  QRef/1 -> Wind Grid-side Converter Controller/1(QRef)
  VIbus/1 -> Wind Grid-side Converter Controller/2(VIBus)
  w/1 -> Machine Converter Control/2(w_sens)
  Machine Converter Control/2(Chopper Control) -> Chopper Control/1
  theta/1 -> Machine Converter Control/3(a_sens)
  Machine Converter Control/1(SM converter control) -> SM converter control/1
  Wind speed/1 -> Machine Converter Control/5(Wind speed)
  vdc/1 -> Machine Converter Control/4(vdc_sens), Wind Grid-side Converter Controller/4(Vdc)
  iPMSM/1 -> Machine Converter Control/1(iabc_sens)
  Wind Grid-side Converter Controller/2(m_abc) -> m_abc/1
  Wind Grid-side Converter Controller/1(FRT) -> Machine Converter Control/6(LVRT)

== system SimscapeCustomComponents_lib/Microgrid and Renewables/Sources/Generator Integrated/Detailed ==
  PRef : Inport
  AVR and Exciter : Subsystem
  "Governor and Prime Mover " : Subsystem  mask(Governor and Prime Mover){pu_speed_reference=pu_speed_reference, droop_percentage=droop_percentage, pu_load_reference_setpoint=pu_load_reference_setpoint, T_G=T_G, T_CH=T_CH, base_torque=base_torque, pu_torque0=pu_torque0}
      mask prompts: pu_speed_reference "Speed reference, (pu)"; droop_percentage "Percentage droop, (%)"; pu_load_reference_setpoint "Load reference setpoint, (pu)"; T_G "Time constant of governor, (s)"; T_CH "Time constant of main inlet volumes and steam chest, (s)"; base_torque "Base torque, (N*m)"; pu_torque0 "Initial torque, (pu)"
      mask help:
      | Implements a synchronous machine governor and prime mover. The prime mover is a non-reheat steam turbine.
      |
      | The input to the block is a per-unit synchronous machine measurement vector.
      |
      | R and C are mechanical rotational ports.
  Inertia : ee_lib/Electromechanical/Mechanical/Machine Inertia  SRated=genRating*1000 V*A  FRated=frequency Hz  nPolePairs=polePairs  inertia_option=2  J=0.5754*200 kg*m^2  H=3.525 s*W/V/A  damper_option=2  D=39.0509 N*m/(rad/s)  pu_D=0.01  initialization_option=2  fMechanical0=60 Hz  fElectrical0=frequency Hz
      settings: InternalSimscapePortConfiguration="{\"Bottom\":[],\"Left\":[{\"id\":\"R\",\"label\":\"R\",\"type\":\"foundation.mechanical.rotational.rotational\"}],\"Right\":[],\"Top\":[]}"
  Machine : ee_lib/Electromechanical/Synchronous/Synchronous Machine Round Rotor  port_option=ee.enum.threePhasePort.composite  SRated=genRating kW  VRated=Vac V  FRated=frequency Hz  nPolePairs=polePairs  param_option=ee.enum.sm.parameterization.standard  fieldCircuitParameterization_option=ee.enum.sm.fieldparameterization.voltage  baseEfd=100 V  baseIfd=1300 A  zero_sequence=ee.enum.park.zerosequence.exclude  axes_param=ee.enum.rotorangle.daxis  Ladu=1.66  Laqu=1.61  L0=0.15  Ll=0.05  Ra=0.03/5  Lfd=0.165  Rfd=0.0006  L1d=0.1713  R1d=0.0284  L1q=0.7252  R1q=0.00619  L2q=0.125  R2q=0.02368  Xl=0.05/5  Xd=1.72/5  Xq=0.79/5  X0=0.06  Xdd=0.13/5  Xqd=0.17/3  Xddd=0.09/5  Xqdd=0.12/5  d_option=ee.enum.circuit.short  Td0d=0.75 s  Tdd=0.03 s  Td0dd=0.03 s  Tddd=0.008 s  q_option=ee.enum.circuit.open  Tq0d=0.6 s  Tqd=0.03 s  Tq0dd=0.02 s  Tqdd=0.008 s  saturation_option=ee.enum.saturation.exclude  saturation_ifd=[0, .48, .76, 1.38, 1.79]  saturation_Vag=[0, .8, 1.08, 1.31, 1.4]  initialization_option=ee.enum.sm.initialization.electrical  source_type=ee.enum.sm.load_flow_source_type.Swing  Vmag0=Vac V  Vang0=0 deg  Pt0=0 A*V  Qt0=0 A*V  minimum_pu=0.95  phase_search_range=[-inf, inf] deg  gmin=1e-4 S  connection_option=ee.enum.Connection.wye  num_q_dampers=2  rotor_offset=-pi / 2 rad  pu_psid_specify=off  pu_psid_priority=None  pu_psid=0  pu_psid_nominal_specify=off  pu_psid_nominal_value=1  pu_psid_nominal_unit=1  pu_psiq_specify=off  pu_psiq_priority=None  pu_psiq=0  pu_psiq_nominal_specify=off  pu_psiq_nominal_value=1  pu_psiq_nominal_unit=1  pu_psifd_specify=off  pu_psifd_priority=None  pu_psifd=0  pu_psifd_nominal_specify=off  pu_psifd_nominal_value=1  pu_psifd_nominal_unit=1  pu_psi1d_specify=off  pu_psi1d_priority=None  pu_psi1d=0  pu_psi1d_nominal_specify=off  pu_psi1d_nominal_value=1  pu_psi1d_nominal_unit=1  pu_psi1q_specify=off  pu_psi1q_priority=None  pu_psi1q=0  pu_psi1q_nominal_specify=off  pu_psi1q_nominal_value=1  pu_psi1q_nominal_unit=1  pu_psi2q_specify=off  pu_psi2q_priority=None  pu_psi2q=0  pu_psi2q_nominal_specify=off  pu_psi2q_nominal_value=1  pu_psi2q_nominal_unit=1  angular_position_diff_specify=off  angular_position_diff_priority=None  angular_position_diff=180 deg  angular_position_diff_nominal_specify=off  angular_position_diff_nominal_value=1  angular_position_diff_nominal_unit=deg  Tmeas=298.15 K  alpha=3.93e-3 1/K  stator_thermal_mass=100 J/K  rotor_thermal_mass=200 J/K  temperatureA_specify=off  temperatureA_priority=High  temperatureA=25 degC  temperatureA_nominal_specify=off  temperatureA_nominal_value=1  temperatureA_nominal_unit=degC  temperatureB_specify=off  temperatureB_priority=High  temperatureB=25 degC  temperatureB_nominal_specify=off  temperatureB_nominal_value=1  temperatureB_nominal_unit=degC  temperatureC_specify=off  temperatureC_priority=High  temperatureC=25 degC  temperatureC_nominal_specify=off  temperatureC_nominal_value=1  temperatureC_nominal_unit=degC  temperatureR_specify=off  temperatureR_priority=High  temperatureR=25 degC  temperatureR_nominal_specify=off  temperatureR_nominal_value=1  temperatureR_nominal_unit=degC
      settings: InternalSimscapePortConfiguration="{\"Bottom\":[],\"Left\":[{\"id\":\"fd_p\",\"label\":\"fd+\",\"type\":\"foundation.electrical.electrical\"},{\"id\":\"fd_n\",\"label\":\"fd-\",\"type\":\"foundation.electrical.electrical\"},{\"id\":\"R\",\"label\":\"R\",\"type\":\"foundation.mechanical.rotational.rotational\"},{\"id\":\"C\",\"label\":\"C\",\"type\":\"foundation.mechanical.rotational.rotational\"}],\"Right\":[{\"id\":\"pu_output\",\"label\":\"pu\",\"type\":\"output\"},{\"id\":\"N\",\"label\":\"~\",\"type\":\"foundation.electrical.three_phase\"}],\"Top\":[]}"
  Measurements : Subsystem
  ~ : PMIOPort  Side=Right
  Bus Element Out : Outport  PortName=Meas  Element=activePower
  BusElementOut : Outport  PortName=Meas  Element=reactivePower
  BusElementOut1 : Outport  PortName=Meas  Element=voltage
  BusElementOut2 : Outport  PortName=Meas  Element=current
  wires:
  PRef/1 -> "Governor and Prime Mover "/1(PRef)
  Measurements/2(Q) -> BusElementOut/1
  Measurements/1(P) -> Bus Element Out/1
  Measurements/3(V) -> BusElementOut1/1
  Measurements/4(I) -> BusElementOut2/1
  connections:
  Machine/LConn2 -- AVR and Exciter/RConn2
  AVR and Exciter/LConn1 -- Machine/RConn1 -- "Governor and Prime Mover "/LConn1
  Inertia/LConn1 -- Machine/LConn3 -- "Governor and Prime Mover "/RConn1
  Machine/LConn4 -- "Governor and Prime Mover "/RConn2
  Machine/LConn1 -- AVR and Exciter/RConn1
  Measurements/LConn1 -- Machine/RConn2
  ~/RConn1 -- Measurements/RConn1

== system SimscapeCustomComponents_lib/Microgrid and Renewables/Sources/Generator Integrated/Simplified ==
  PRef : Inport
  Electrical Reference : fl_lib/Electrical/Electrical Elements/Electrical Reference
  Exciter : Subsystem
  Machine : ee_lib/Electromechanical/Synchronous/Synchronous Machine Round Rotor  port_option=ee.enum.threePhasePort.composite  SRated=genRating kW  VRated=Vac V  FRated=frequency Hz  nPolePairs=polePairs  param_option=ee.enum.sm.parameterization.standard  fieldCircuitParameterization_option=ee.enum.sm.fieldparameterization.voltage  baseEfd=100 V  baseIfd=1300 A  zero_sequence=ee.enum.park.zerosequence.exclude  axes_param=ee.enum.rotorangle.daxis  Ladu=1.66  Laqu=1.61  L0=0.15  Ll=0.05  Ra=0.03/5  Lfd=0.165  Rfd=0.0006  L1d=0.1713  R1d=0.0284  L1q=0.7252  R1q=0.00619  L2q=0.125  R2q=0.02368  Xl=0.05/5  Xd=1.72/5  Xq=0.79/5  X0=0.06  Xdd=0.13/5  Xqd=0.17/3  Xddd=0.09/5  Xqdd=0.12/5  d_option=ee.enum.circuit.short  Td0d=0.75 s  Tdd=0.03 s  Td0dd=0.03 s  Tddd=0.008 s  q_option=ee.enum.circuit.open  Tq0d=0.6 s  Tqd=0.03 s  Tq0dd=0.02 s  Tqdd=0.008 s  saturation_option=ee.enum.saturation.exclude  saturation_ifd=[0, .48, .76, 1.38, 1.79]  saturation_Vag=[0, .8, 1.08, 1.31, 1.4]  initialization_option=ee.enum.sm.initialization.electrical  source_type=ee.enum.sm.load_flow_source_type.Swing  Vmag0=Vac V  Vang0=0 deg  Pt0=0 A*V  Qt0=0 A*V  minimum_pu=0.95  phase_search_range=[-inf, inf] deg  gmin=1e-4 S  connection_option=ee.enum.Connection.wye  num_q_dampers=2  rotor_offset=-pi / 2 rad  pu_psid_specify=off  pu_psid_priority=None  pu_psid=0  pu_psid_nominal_specify=off  pu_psid_nominal_value=1  pu_psid_nominal_unit=1  pu_psiq_specify=off  pu_psiq_priority=None  pu_psiq=0  pu_psiq_nominal_specify=off  pu_psiq_nominal_value=1  pu_psiq_nominal_unit=1  pu_psifd_specify=off  pu_psifd_priority=None  pu_psifd=0  pu_psifd_nominal_specify=off  pu_psifd_nominal_value=1  pu_psifd_nominal_unit=1  pu_psi1d_specify=off  pu_psi1d_priority=None  pu_psi1d=0  pu_psi1d_nominal_specify=off  pu_psi1d_nominal_value=1  pu_psi1d_nominal_unit=1  pu_psi1q_specify=off  pu_psi1q_priority=None  pu_psi1q=0  pu_psi1q_nominal_specify=off  pu_psi1q_nominal_value=1  pu_psi1q_nominal_unit=1  pu_psi2q_specify=off  pu_psi2q_priority=None  pu_psi2q=0  pu_psi2q_nominal_specify=off  pu_psi2q_nominal_value=1  pu_psi2q_nominal_unit=1  angular_position_diff_specify=off  angular_position_diff_priority=None  angular_position_diff=180 deg  angular_position_diff_nominal_specify=off  angular_position_diff_nominal_value=1  angular_position_diff_nominal_unit=deg  Tmeas=298.15 K  alpha=3.93e-3 1/K  stator_thermal_mass=100 J/K  rotor_thermal_mass=200 J/K  temperatureA_specify=off  temperatureA_priority=High  temperatureA=25 degC  temperatureA_nominal_specify=off  temperatureA_nominal_value=1  temperatureA_nominal_unit=degC  temperatureB_specify=off  temperatureB_priority=High  temperatureB=25 degC  temperatureB_nominal_specify=off  temperatureB_nominal_value=1  temperatureB_nominal_unit=degC  temperatureC_specify=off  temperatureC_priority=High  temperatureC=25 degC  temperatureC_nominal_specify=off  temperatureC_nominal_value=1  temperatureC_nominal_unit=degC  temperatureR_specify=off  temperatureR_priority=High  temperatureR=25 degC  temperatureR_nominal_specify=off  temperatureR_nominal_value=1  temperatureR_nominal_unit=degC
      settings: InternalSimscapePortConfiguration="{\"Bottom\":[],\"Left\":[{\"id\":\"fd_p\",\"label\":\"fd+\",\"type\":\"foundation.electrical.electrical\"},{\"id\":\"fd_n\",\"label\":\"fd-\",\"type\":\"foundation.electrical.electrical\"},{\"id\":\"R\",\"label\":\"R\",\"type\":\"foundation.mechanical.rotational.rotational\"},{\"id\":\"C\",\"label\":\"C\",\"type\":\"foundation.mechanical.rotational.rotational\"}],\"Right\":[{\"id\":\"pu_output\",\"label\":\"pu\",\"type\":\"output\"},{\"id\":\"N\",\"label\":\"~\",\"type\":\"foundation.electrical.three_phase\"}],\"Top\":[]}"
  Machine Inertia : ee_lib/Electromechanical/Mechanical/Machine Inertia  SRated=genRating*1000 V*A  FRated=frequency Hz  nPolePairs=polePairs  inertia_option=1  J=0.5754 kg*m^2  H=3.525 s*W/V/A  damper_option=2  D=39.0509 N*m/(rad/s)  pu_D=0.01  initialization_option=2  fMechanical0=60 Hz  fElectrical0=60 Hz
      settings: InternalSimscapePortConfiguration="{\"Bottom\":[],\"Left\":[{\"id\":\"R\",\"label\":\"R\",\"type\":\"foundation.mechanical.rotational.rotational\"}],\"Right\":[],\"Top\":[]}"
  Measurements : Subsystem
  Prime Mover : Subsystem
  ~ : PMIOPort  Side=Right
  Bus Element Out : Outport  PortName=Meas  Element=activePower
  BusElementOut : Outport  PortName=Meas  Element=reactivePower
  BusElementOut1 : Outport  PortName=Meas  Element=voltage
  BusElementOut2 : Outport  PortName=Meas  Element=current
  wires:
  PRef/1 -> Prime Mover/1(PRef)
  Measurements/4(I) -> BusElementOut2/1
  Measurements/3(V) -> BusElementOut1/1
  Measurements/1(P) -> Bus Element Out/1
  Measurements/2(Q) -> BusElementOut/1
  connections:
  Exciter/RConn2 -- Machine/LConn2 -- Electrical Reference/LConn1
  Machine Inertia/LConn1 -- Prime Mover/RConn1 -- Machine/LConn3
  Exciter/RConn1 -- Machine/LConn1
  Prime Mover/RConn2 -- Machine/LConn4
  ~/RConn1 -- Measurements/RConn1
  Measurements/LConn1 -- Machine/RConn2

== system SimscapeCustomComponents_lib/Microgrid and Renewables/Sources/Solar Plant/Converter ==
  mabc : Inport
  Average : Subsystem  VariantControl=Average
  Switching : Subsystem  VariantControl=Switching
  + : PMIOPort  Side=Left
  - : PMIOPort  Port=2  Side=Left
  ~ : PMIOPort  Port=3  Side=Right

== system SimscapeCustomComponents_lib/Microgrid and Renewables/Sources/Solar Plant Integrated/Detailed ==
  Ir : Inport
  T : Inport  Port=2
  Pref : Inport  Port=3
  Qref : Inport  Port=4
  Mode : Inport  Port=5
  L Filter2 : ee_lib/Passive/RLC Assemblies/RLC (Three-Phase)  port_option=ee.enum.threePhasePort.composite  component_structure=ee.enum.rlc.structure.SeriesRL  R=filterResistance Ohm  L=filterInductance H  C=1e-6 F  R_parasitic=0 Ohm  G_parasitic=0 1/Ohm  IL_specify=on  IL_priority=None  IL=[0, 0, 0] A  IL_nominal_specify=off  IL_nominal_value=1  IL_nominal_unit=A  VC_specify=off  VC_priority=High  VC=[0, 0, 0] V  VC_nominal_specify=off  VC_nominal_value=1  VC_nominal_unit=V
      settings: InternalSimscapePortConfiguration="{\"Bottom\":[],\"Left\":[{\"id\":\"N1\",\"label\":\"~1\",\"type\":\"foundation.electrical.three_phase\"}],\"Right\":[{\"id\":\"N2\",\"label\":\"~2\",\"type\":\"foundation.electrical.three_phase\"}],\"Top\":[]}"
  Measurements : Subsystem
  PV Plant & Controller : Subsystem
  Terminator : Terminator
  ~ : PMIOPort  Side=Right
  Out Bus Element23 : Outport  PortName=Meas  Element=activePower
  Out Bus Element1 : Outport  PortName=Meas  Element=reactivePower
  Out Bus Element2 : Outport  PortName=Meas  Element=voltage
  Out Bus Element3 : Outport  PortName=Meas  Element=current
  wires:
  Mode/1 -> PV Plant & Controller/6(Mode)
  Pref/1 -> PV Plant & Controller/2(Pref)
  T/1 -> Terminator/1
  Measurements/1(P) -> Out Bus Element23/1
  Measurements/3(V) -> PV Plant & Controller/4(Vabc), Out Bus Element2/1
  Ir/1 -> PV Plant & Controller/1(Insolation)
  Qref/1 -> PV Plant & Controller/3(Qref)
  Measurements/4(I) -> PV Plant & Controller/5(Iabc), Out Bus Element3/1
  Measurements/2(Q) -> Out Bus Element1/1
  connections:
  Measurements/RConn1 -- ~/RConn1
  L Filter2/LConn1 -- PV Plant & Controller/RConn1
  L Filter2/RConn1 -- Measurements/LConn1

== system SimscapeCustomComponents_lib/Microgrid and Renewables/Sources/Solar Plant Integrated/Simplified ==
  Ir : Inport
  T : Inport  Port=2
  Pref : Inport  Port=3
  Qref : Inport  Port=4
  Mode : Inport  Port=5
  Measurements : Subsystem
  Simulink-PS Converter{,1..4} (5 alike) : nesl_utility/Simulink-PS Converter  PhysicalDomain=network_engine_domain  SubClassName=ps_input  LeftPortType=input  RightPortType=output  PseudoPeriodic=off  Frequencies=[]  NoiseDistribution=none  NoiseParameters=[]  Unit=1  AffineConversion=off  FilteringAndDerivatives=provide  SimscapeFilterOrder=1  InputFilterTimeConstant=0.001  UdotUserProvided=0
  solar_plant : microgridRenewables_lib/solar_plant  port_option=ee.enum.threePhasePort.composite  FRated=60 Hz  VRated=415 V  PlantRating=100e3 W  modelling_option=ModellingOption.powerReference  Vdc=1000 V  IMaxPU=1.2  efficiency=100  IrRef=100 W/m^2  T=298 K  PVTech=PanelTechnology.polycrystallinePanel  PanelRating=100 W  VocRef=100 V  IscRef=100 A  alpha=0.005 1/K  beta=-0.005 1/K  delta=0.111
      settings: InternalSimscapePortConfiguration="{\"Bottom\":[],\"Left\":[{\"id\":\"Ir\",\"label\":\"Ir\",\"type\":\"input\"},{\"id\":\"Tsim\",\"label\":\"T\",\"type\":\"input\"},{\"id\":\"Mode\",\"label\":\"Mode\",\"type\":\"input\"},{\"id\":\"Pref\",\"label\":\"Pref\",\"type\":\"input\"},{\"id\":\"Qref\",\"label\":\"Qref\",\"type\":\"input\"}],\"Right\":[{\"id\":\"N\",\"label\":\"~\",\"type\":\"foundation.electrical.three_phase\"},{\"id\":\"l\",\"label\":\"l\",\"type\":\"output\"},{\"id\":\"p\",\"label\":\"p\",\"type\":\"output\"}],\"Top\":[]}"
  ~ : PMIOPort  Side=Right
  Bus Element Out : Outport  PortName=Meas  Element=activePower
  BusElementOut : Outport  PortName=Meas  Element=reactivePower
  BusElementOut1 : Outport  PortName=Meas  Element=voltage
  BusElementOut2 : Outport  PortName=Meas  Element=current
  wires:
  Mode/1 -> Simulink-PS Converter4/1
  Qref/1 -> Simulink-PS Converter3/1
  Pref/1 -> Simulink-PS Converter2/1
  T/1 -> Simulink-PS Converter1/1
  Ir/1 -> Simulink-PS Converter/1
  Measurements/1(P) -> Bus Element Out/1
  Measurements/2(Q) -> BusElementOut/1
  Measurements/3(V) -> BusElementOut1/1
  Measurements/4(I) -> BusElementOut2/1
  connections:
  solar_plant/LConn4 -- Simulink-PS Converter2/RConn1
  solar_plant/LConn2 -- Simulink-PS Converter1/RConn1
  solar_plant/LConn1 -- Simulink-PS Converter/RConn1
  solar_plant/RConn1 -- Measurements/LConn1
  ~/RConn1 -- Measurements/RConn1
  solar_plant/LConn3 -- Simulink-PS Converter4/RConn1
  solar_plant/LConn5 -- Simulink-PS Converter3/RConn1

== system SimscapeCustomComponents_lib/Microgrid and Renewables/Sources/Wind Plant/Back-to-Back Converters ==
  Chopper : Inport
  SM_ref : Inport  Port=2
  Grid_ref : Inport  Port=3
  Average : Subsystem  VariantControl=Average
  Switching : Subsystem  VariantControl=Switching
  In : PMIOPort  Side=Left
  ~ : PMIOPort  Port=2  Side=Right
  Vdc : Outport

== system SimscapeCustomComponents_lib/Microgrid and Renewables/Sources/Wind Plant Integrated/Detailed ==
  LVRT : Inport
  QRef : Inport  Port=2
  WindSpeed : Inport  Port=3
  Constant : Constant  Value=0
  L Filter : ee_lib/Passive/RLC Assemblies/RLC (Three-Phase)  port_option=ee.enum.threePhasePort.composite  component_structure=ee.enum.rlc.structure.L  R=1e-3 Ohm  L=filterInductance H  C=1e-6 F  R_parasitic=0 Ohm  G_parasitic=0 1/Ohm  IL_specify=off  IL_priority=High  IL=[0, 0, 0] A  IL_nominal_specify=off  IL_nominal_value=1  IL_nominal_unit=A  VC_specify=off  VC_priority=High  VC=[0, 0, 0] V  VC_nominal_specify=off  VC_nominal_value=1  VC_nominal_unit=V
      settings: InternalSimscapePortConfiguration="{\"Bottom\":[],\"Left\":[{\"id\":\"N1\",\"label\":\"~1\",\"type\":\"foundation.electrical.three_phase\"}],\"Right\":[{\"id\":\"N2\",\"label\":\"~2\",\"type\":\"foundation.electrical.three_phase\"}],\"Top\":[]}"
  Measurements : Subsystem
  PLL : Subsystem
  Wind Turbine and Converters : Subsystem
  ~ : PMIOPort  Side=Right
  Out Bus Element : Outport  PortName=Meas  Element=activePower
  BusElementOut : Outport  PortName=Meas  Element=reactivePower
  BusElementOut1 : Outport  PortName=Meas  Element=voltage
  BusElementOut2 : Outport  PortName=Meas  Element=current
  wires:
  LVRT/1 -> Wind Turbine and Converters/3(LVRT)
  WindSpeed/1 -> Wind Turbine and Converters/2(Wind_speed)
  QRef/1 -> Wind Turbine and Converters/4(QRef)
  PLL/1(VI) -> Wind Turbine and Converters/5(VIBus)
  Constant/1 -> Wind Turbine and Converters/1(pitch)
  Measurements/1(P) -> Out Bus Element/1
  Measurements/2(Q) -> BusElementOut/1
  Measurements/3(V) -> BusElementOut1/1, PLL/1(V)
  Measurements/4(I) -> BusElementOut2/1, PLL/2(I)
  connections:
  L Filter/LConn1 -- Wind Turbine and Converters/RConn1
  L Filter/RConn1 -- Measurements/LConn1
  ~/RConn1 -- Measurements/RConn1
